simulink model "left"  (R2016b)
settings: Solver=VariableStepAuto  StartTime=0.0  StopTime=10.0  RelTol=1e-3
libraries: TLMLib x1
settings Model: Creator=robbr48  LastModifiedBy=robbr48

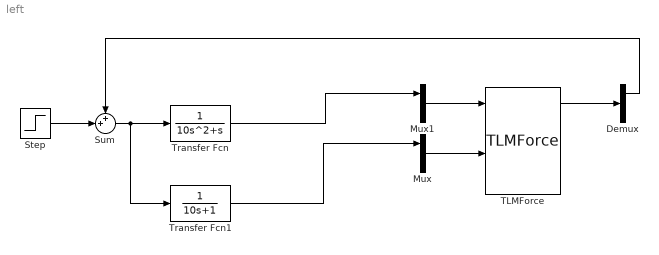
== system left ==
  Demux : Demux  Outputs=3
  Mux : Mux  Inputs=3
  Mux1 : Mux  Inputs=3
  Step : Step  After=100  SampleTime=0
  Sum : Sum  Inputs=++|
  TLMForce : TLMLib/TLMForce
  Transfer Fcn : TransferFcn  Denominator=[10 1 0]
  Transfer Fcn1 : TransferFcn  Denominator=[10 1]
  wires:
  TLMForce/1 -> Demux/1
  Mux/1 -> TLMForce/3
  Mux1/1 -> TLMForce/1
  Sum/1 -> Transfer Fcn1/1, Transfer Fcn/1
  Transfer Fcn1/1 -> Mux/1
  Transfer Fcn/1 -> Mux1/1
  Step/1 -> Sum/2
  Demux/1 -> Sum/1
